simulink library "WaterRunner_lib"  (Simulink 7.9)
settings: Solver=ode45  StartTime=0.0  StopTime=10.0  RelTol=1e-3
values from neighbouring files (symbols this model uses):
  water_level = u(6)    [water_model.m]
undefined symbols (not defined in the file or in its folder): frame_inertia, frame_mass, initRobHeight, L2_inertia, L2_mass, L3_inertia, L3_mass, L4_inertia, L4_mass, median_speed, motor_inertia, motor_mass, mu_slide, mu_stick, phase_delay, pulse_amplitude, pulse_df, pulse_period, speed, switch_angle, Tail_inertia, Tail_mass, tau, V_H
libraries: mblibv1 x42, simulink x2
settings Model: Creator=Metti  LastModifiedBy=nitisht

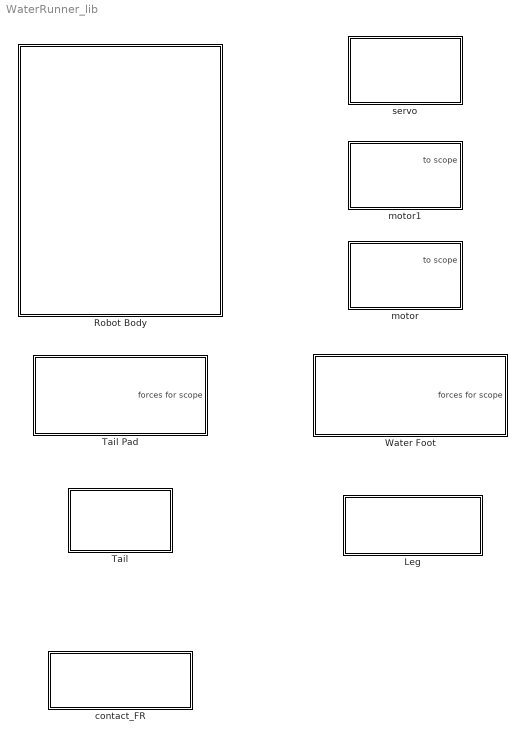
== system WaterRunner_lib ==
  Leg : Subsystem
      mask Description: mask for leg
  Robot Body : Subsystem  mask{initRobHeight=initRobHeight}
      mask prompts: initRobHeight "height"
  Tail : Subsystem
  Tail Pad : Subsystem
  Water Foot : Subsystem
  contact_FR : Subsystem
  motor : Subsystem  mask{variableName=work, ic_angle=0}
      mask prompts: variableName "Variable Name for Work"; ic_angle "initial angle"
      mask init:
      | set_param([gcb '/To Workspace'],'VariableName',variableName)
  motor1 : Subsystem  mask{speed=speed, X0=0, VariableName=work}
      mask prompts: speed "Rotation Speed:"; X0 "Initial output:"; VariableName "Variable name for Work:"
  servo : Subsystem  mask{tail_angle=speed, VariableName=work}
      mask prompts: tail_angle "Tail angle"; VariableName "Variable name for Work:"

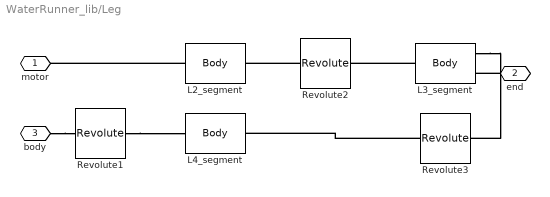
== system WaterRunner_lib/Leg ==
  L2_segment : mblibv1/Bodies/Body  LConnTagsString=CS1  RConnTagsString=CS2  UpdateFromCAD=off  DialogClass=MechanicalBodyBlock  Mass=L2_mass  MassUnits=kg  InertiaUnits=kg*m^2  Inertia=L2_inertia  Shape=Cylinder  ShapeDims=[1 1]  ShapeUnits=m  ShapeUse=false  Density=1  DensityUnits=kg/m^3  DensityUse=false  GraphicsMode=CONVHULL  BodyColorSelMode=COLORPALETTE  BodyColor=[0 0 0]  AttachedToCS=CG  CG=Left$CG$L2_CG$CS1$CS1$m$[0 0 0]$Euler X-Y-Z$deg$WORLD$false$none  WorkingFrames=Left$CS1$L2_CS1$Adjoining$Adjoining$m$[0 0 0]$Euler X-Y-Z$deg$WORLD$true$none#Right$CS2$L2_CS2$CS1$CS1$m$[0 0 0]$Euler X-Y-Z$deg$WORLD$true$none  CGPos=L2_CG  CGRot=[0 0 0]  CS0Pos=[]  CS0Rot=[]  CS1Pos=L2_CS1  CS1Rot=[0 0 0]  CS2Pos=L2_CS2  CS2Rot=[0 0 0]  CS3Pos=[]  CS3Rot=[]  CS4Pos=[]  CS4Rot=[]  CS5Pos=[]  CS5Rot=[]  CS6Pos=[]  CS6Rot=[]  CS7Pos=[]  CS7Rot=[]  CS8Pos=[]  CS8Rot=[]  CS9Pos=[]  CS9Rot=[]  CS10Pos=[]  CS10Rot=[]  CS11Pos=[]  CS11Rot=[]  CS12Pos=[]  CS12Rot=[]  CS13Pos=[]  CS13Rot=[]  CS14Pos=[]  CS14Rot=[]  CS15Pos=[]  CS15Rot=[]  CS16Pos=[]  CS16Rot=[]  CS17Pos=[]  CS17Rot=[]  CS18Pos=[]  CS18Rot=[]  CS19Pos=[]  CS19Rot=[]  CS20Pos=[]  CS20Rot=[]
  L3_segment : mblibv1/Bodies/Body  LConnTagsString=CS1  RConnTagsString=CS2|CS3  UpdateFromCAD=off  DialogClass=MechanicalBodyBlock  Mass=L3_mass  MassUnits=kg  InertiaUnits=kg*m^2  Inertia=L3_inertia  Shape=Cylinder  ShapeDims=[1 1]  ShapeUnits=m  ShapeUse=false  Density=1  DensityUnits=kg/m^3  DensityUse=false  GraphicsMode=CONVHULL  BodyColorSelMode=COLORPALETTE  BodyColor=[0 0 0]  AttachedToCS=CG  CG=Left$CG$L3_CG$CS1$CS1$m$[0 0 0]$Euler X-Y-Z$rad$CS1$false$none  WorkingFrames=Left$CS1$L3_CS1$Adjoining$Adjoining$m$L3_ori$Euler X-Y-Z$rad$Adjoining$true$none#Right$CS2$L3_CS2$CS1$CS1$m$[0 0 0]$Euler X-Y-Z$rad$CS1$true$none#Right$CS3$L3_CS3$CS1$CS1$m$[0 0 0]$Euler X-Y-Z$rad$CS1$true$none  CGPos=L3_CG  CGRot=[0 0 0]  CS0Pos=[]  CS0Rot=[]  CS1Pos=L3_CS1  CS1Rot=L3_ori  CS2Pos=L3_CS2  CS2Rot=[0 0 0]  CS3Pos=L3_CS3  CS3Rot=[0 0 0]  CS4Pos=[]  CS4Rot=[]  CS5Pos=[]  CS5Rot=[]  CS6Pos=[]  CS6Rot=[]  CS7Pos=[]  CS7Rot=[]  CS8Pos=[]  CS8Rot=[]  CS9Pos=[]  CS9Rot=[]  CS10Pos=[]  CS10Rot=[]  CS11Pos=[]  CS11Rot=[]  CS12Pos=[]  CS12Rot=[]  CS13Pos=[]  CS13Rot=[]  CS14Pos=[]  CS14Rot=[]  CS15Pos=[]  CS15Rot=[]  CS16Pos=[]  CS16Rot=[]  CS17Pos=[]  CS17Rot=[]  CS18Pos=[]  CS18Rot=[]  CS19Pos=[]  CS19Rot=[]  CS20Pos=[]  CS20Rot=[]
  L4_segment : mblibv1/Bodies/Body  LConnTagsString=CS1  RConnTagsString=CS2  UpdateFromCAD=off  DialogClass=MechanicalBodyBlock  Mass=L4_mass  MassUnits=kg  InertiaUnits=kg*m^2  Inertia=L4_inertia  Shape=Cylinder  ShapeDims=[1 1]  ShapeUnits=m  ShapeUse=false  Density=1  DensityUnits=kg/m^3  DensityUse=false  GraphicsMode=CONVHULL  BodyColorSelMode=COLORPALETTE  BodyColor=[0 0 0]  AttachedToCS=CG  CG=Left$CG$L4_CG$CS1$CS1$m$[0 0 0]$Euler X-Y-Z$rad$CS1$false$none  WorkingFrames=Left$CS1$L4_CS1$Adjoining$Adjoining$m$L4_ori$Euler X-Y-Z$rad$Adjoining$true$none#Right$CS2$L4_CS2$CS1$CS1$m$[0 0 0]$Euler X-Y-Z$rad$CS1$true$none  CGPos=L4_CG  CGRot=[0 0 0]  CS0Pos=[]  CS0Rot=[]  CS1Pos=L4_CS1  CS1Rot=L4_ori  CS2Pos=L4_CS2  CS2Rot=[0 0 0]  CS3Pos=[]  CS3Rot=[]  CS4Pos=[]  CS4Rot=[]  CS5Pos=[]  CS5Rot=[]  CS6Pos=[]  CS6Rot=[]  CS7Pos=[]  CS7Rot=[]  CS8Pos=[]  CS8Rot=[]  CS9Pos=[]  CS9Rot=[]  CS10Pos=[]  CS10Rot=[]  CS11Pos=[]  CS11Rot=[]  CS12Pos=[]  CS12Rot=[]  CS13Pos=[]  CS13Rot=[]  CS14Pos=[]  CS14Rot=[]  CS15Pos=[]  CS15Rot=[]  CS16Pos=[]  CS16Rot=[]  CS17Pos=[]  CS17Rot=[]  CS18Pos=[]  CS18Rot=[]  CS19Pos=[]  CS19Rot=[]  CS20Pos=[]  CS20Rot=[]
  Revolute1 : mblibv1/Joints/Revolute  LConnTagsString=__newl0  RConnTagsString=__newr0  UpdateFromCAD=off  NumSAPorts=0  CutJoint=off  MarkAsCut=off  Primitives=prismatic  PrimitiveProps=R1$WORLD$[0 0 1]$revolute  DialogClass=JointBlock  R1Axis=[0 0 1]
  Revolute2 : mblibv1/Joints/Revolute  LConnTagsString=__newl0  RConnTagsString=__newr0  UpdateFromCAD=off  NumSAPorts=0  CutJoint=off  MarkAsCut=off  Primitives=prismatic  PrimitiveProps=R1$WORLD$[0 0 1]$revolute  DialogClass=JointBlock  R1Axis=[0 0 1]
  Revolute3 : mblibv1/Joints/Revolute  LConnTagsString=__newl0  RConnTagsString=__newr0  UpdateFromCAD=off  NumSAPorts=0  CutJoint=on  MarkAsCut=off  Primitives=prismatic  PrimitiveProps=R1$World$[0 0 1]$revolute  DialogClass=JointBlock  R1Axis=[0 0 1]
  motor : PMIOPort  Port=1  Side=Left
  end : PMIOPort  Port=2  Side=Right
  body : PMIOPort  Port=3  Side=Left
  connections:
  body/RConn1 -- Revolute1/LConn1
  end/RConn1 -- L3_segment/RConn2
  Revolute3/LConn1 -- L4_segment/RConn1
  Revolute1/RConn1 -- L4_segment/LConn1
  L3_segment/RConn1 -- Revolute3/RConn1
  L3_segment/LConn1 -- Revolute2/RConn1
  Revolute2/LConn1 -- L2_segment/RConn1
  L2_segment/LConn1 -- motor/RConn1

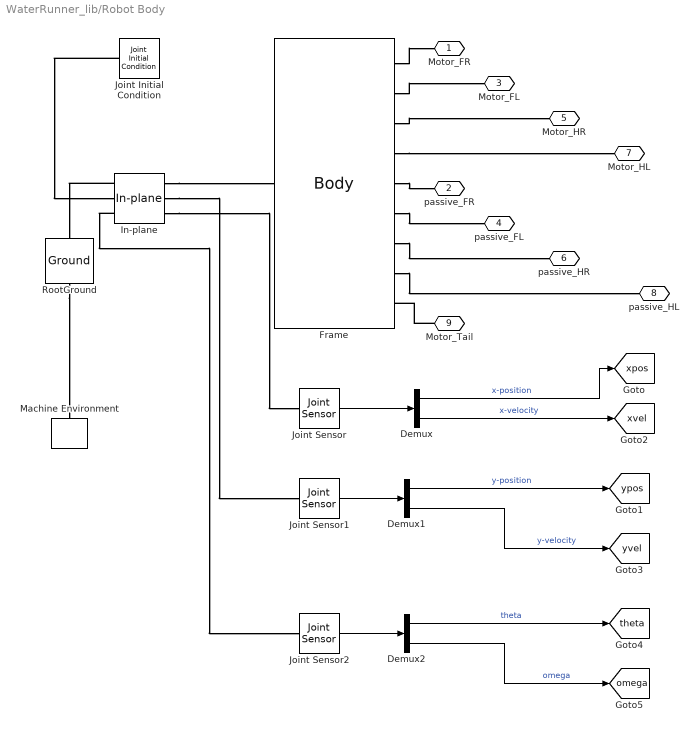
== system WaterRunner_lib/Robot Body ==
  Demux : Demux  Outputs=2
  Demux1 : Demux  Outputs=2
  Demux2 : Demux  Outputs=2
  Frame : mblibv1/Bodies/Body  LConnTagsString=CS1  RConnTagsString=CS6|CS7|CS8|CS9|CS10|CS11|CS12|CS13|CS14  UpdateFromCAD=off  DialogClass=MechanicalBodyBlock  Mass=frame_mass  MassUnits=kg  InertiaUnits=kg*m^2  Inertia=frame_inertia  Shape=Cylinder  ShapeDims=[1 1]  ShapeUnits=m  ShapeUse=false  Density=1  DensityUnits=kg/m^3  DensityUse=false  GraphicsMode=CONVHULL  BodyColorSelMode=COLORPALETTE  BodyColor=[0 0 1]  AttachedToCS=CG  CG=Left$CG$frame_CG$WORLD$WORLD$m$[0 0 0]$Euler X-Y-Z$deg$WORLD$false$none  WorkingFrames=Left$CS1$frame_CA$World$World$m$[0 0 0]$Euler X-Y-Z$deg$WORLD$true$none#Right$CS2$frame_FR$World$World$m$[0 0 0]$Euler X-Y-Z$deg$WORLD$false$none#Right$CS4$frame_FL$World$World$m$[0 0 0]$Euler X-Y-Z$deg$WORLD$false$none#Right$CS3$frame_HR$World$World$m$[0 0 0]$Euler X-Y-Z$deg$WORLD$false$none#Right$CS5$frame_HL$WORLD$WORLD$m$[0 0 0]$Euler X-Y-Z$deg$WORLD$false$none#Right$CS6$frame_motor_FR$WORLD$WORLD$m$[0 0 0]$Euler X-Y-Z$deg$WORLD$true$none#Right$CS7$frame_motor_FL$WORLD$WORLD$m$[0 0 0]$Euler X-Y-Z$deg$WORLD$true$none#Right$CS8$frame_motor_HR$WORLD$WORLD$m$[0 0 0]$Euler X-Y-Z$deg$WORLD$true$none#Right$CS9$frame_motor_HL$WORLD$WORLD$m$[0 0 0]$Euler X-Y-Z$deg$WORLD$true$none#Right$CS10$frame_passive_FR$WORLD$WORLD$m$[0 0 0]$Euler X-Y-Z$deg$WORLD$true$none#Right$CS11$frame_passive_FL$WORLD$WORLD$m$[0 0 0]$Euler X-Y-Z$deg$WORLD$true$none#Right$CS12$frame_passive_HR$WORLD$WORLD$m$[0 0 0]$Euler X-Y-Z$deg$WORLD$true$none#Right$CS13$frame_passive_HL$WORLD$WORLD$m$[0 0 0]$Euler X-Y-Z$deg$WORLD$true$none#Right$CS14$frame_motor_Tail$WORLD$WORLD$m$[0 0 0]$Euler X-Y-Z$deg$WORLD$true$none  CGPos=frame_CG  CGRot=[0 0 0]  CS0Pos=[]  CS0Rot=[]  CS1Pos=frame_CA  CS1Rot=[0 0 0]  CS2Pos=frame_FR  CS2Rot=[0 0 0]  CS3Pos=frame_HR  CS3Rot=[0 0 0]  CS4Pos=frame_FL  CS4Rot=[0 0 0]  CS5Pos=frame_HL  CS5Rot=[0 0 0]  CS6Pos=frame_motor_FR  CS6Rot=[0 0 0]  CS7Pos=frame_motor_FL  CS7Rot=[0 0 0]  CS8Pos=frame_motor_HR  CS8Rot=[0 0 0]  CS9Pos=frame_motor_HL  CS9Rot=[0 0 0]  CS10Pos=frame_passive_FR  CS10Rot=[0 0 0]  CS11Pos=frame_passive_FL  CS11Rot=[0 0 0]  CS12Pos=frame_passive_HR  CS12Rot=[0 0 0]  CS13Pos=frame_passive_HL  CS13Rot=[0 0 0]  CS14Pos=frame_motor_Tail  CS14Rot=[0 0 0]  CS15Pos=[]  CS15Rot=[]  CS16Pos=[]  CS16Rot=[]  CS17Pos=[]  CS17Rot=[]  CS18Pos=[]  CS18Rot=[]  CS19Pos=[]  CS19Rot=[]  CS20Pos=[]  CS20Rot=[]
  In-plane : mblibv1/Joints/In-plane  LConnTagsString=__newl0|SA1|SA2  RConnTagsString=__newr0|SA1|SA2  UpdateFromCAD=off  NumSAPorts=4  CutJoint=off  MarkAsCut=off  Primitives=prismatic  PrimitiveProps=P1$World$[1 0 0]$prismatic#P2$World$[0 1 0]$prismatic  DialogClass=JointBlock  P1Axis=[1 0 0]  P2Axis=[0 1 0]
  Joint Initial Condition : mblibv1/Sensors &  Actuators/Joint Initial Condition  UpdateFromCAD=off  LeftPortType=blob  RightPortType=blob  PhysicalDomain=mechanical  DialogClass=InitialConditionBlock  InitialConditions=P1$true$0$m$deg$0$m/s$deg/s#P2$true$initRobHeight$m$deg$0$m/s$deg/s#P3$false$0$m$deg$0$m/s$deg/s#R1$false$0$m$rad$0$m/s$rad/s#R2$false$0$m$deg$0$m/s$deg/s#R3$false$0$m$deg$0$m/s$deg/s#S$false$0$m$deg$0$m/s$deg/s  P1PIC=0  P1VIC=0  P2PIC=initRobHeight  P2VIC=0  P3PIC=0  P3VIC=0  R1PIC=0  R1VIC=0  R2PIC=0  R2VIC=0  R3PIC=0  R3VIC=0  SPIC=0  SVIC=0
  Joint Sensor : mblibv1/Sensors &  Actuators/Joint Sensor  UpdateFromCAD=off  PhysicalDomain=Mechanical  PortType=blob  Muxed=on  Pose=off  Angle=on  AngleUnits=deg  ArcVelocity=off  ArcVelocityUnits=deg/s  ArcAcceleration=off  ArcAccelerationUnits=deg/s^2  CoordPosition=on  CoordPositionUnits=m  Velocity=on  VelocityUnits=m/s  Acceleration=off  AccelerationUnits=m/s^2  Quaternion=on  QuaternionDT=off  QuaternionDDT=off  QuaternionUnits=off  OutputVector=[1]  ActiveIO=off  Width=2  DialogClass=MechanicalSensorBlock  Primitive=P1  Force=off  ForceUnits=N  Torque=off  TorqueUnits=N*m  ReferenceFrame=Absolute (World)  ReactionSensedSide=Base  ReactionReferenceFrame=Absolute (World)  ReactionForce=off  ReactionForceUnits=N  ReactionMoment=off  ReactionMomentUnits=N*m
  Joint Sensor1 : mblibv1/Sensors &  Actuators/Joint Sensor  UpdateFromCAD=off  PhysicalDomain=Mechanical  PortType=blob  Muxed=on  Pose=off  Angle=on  AngleUnits=deg  ArcVelocity=off  ArcVelocityUnits=deg/s  ArcAcceleration=off  ArcAccelerationUnits=deg/s^2  CoordPosition=on  CoordPositionUnits=m  Velocity=on  VelocityUnits=m/s  Acceleration=off  AccelerationUnits=m/s^2  Quaternion=on  QuaternionDT=off  QuaternionDDT=off  QuaternionUnits=off  OutputVector=[1]  ActiveIO=off  Width=2  DialogClass=MechanicalSensorBlock  Primitive=P2  Force=off  ForceUnits=N  Torque=off  TorqueUnits=N*m  ReferenceFrame=Absolute (World)  ReactionSensedSide=Base  ReactionReferenceFrame=Absolute (World)  ReactionForce=off  ReactionForceUnits=N  ReactionMoment=off  ReactionMomentUnits=N*m
  Joint Sensor2 : mblibv1/Sensors &  Actuators/Joint Sensor  UpdateFromCAD=off  PhysicalDomain=Mechanical  PortType=blob  Muxed=on  Pose=off  Angle=on  AngleUnits=rad  ArcVelocity=on  ArcVelocityUnits=rad/s  ArcAcceleration=off  ArcAccelerationUnits=deg/s^2  CoordPosition=on  CoordPositionUnits=m  Velocity=on  VelocityUnits=m/s  Acceleration=off  AccelerationUnits=m/s^2  Quaternion=on  QuaternionDT=off  QuaternionDDT=off  QuaternionUnits=off  OutputVector=[1]  ActiveIO=off  Width=1  DialogClass=MechanicalSensorBlock  Primitive=P2  Force=off  ForceUnits=N  Torque=off  TorqueUnits=N*m  ReferenceFrame=Absolute (World)  ReactionSensedSide=Base  ReactionReferenceFrame=Absolute (World)  ReactionForce=off  ReactionForceUnits=N  ReactionMoment=off  ReactionMomentUnits=N*m
  Machine Environment : mblibv1/Bodies/Machine Environment  PortType=env  PhysicalDomain=Mechanical  DialogTemplateClass=MECH.MachineEnvironment  SyncWhenCopied=off  Gravity=[0 -9.81 0]  GravityUnits=m/s^2  GravityAsSignal=off  Dimensionality=Auto-detect  AnalysisType=Forward dynamics  LinearAssemblyTolerance=1e-3  LinearAssemblyToleranceUnits=m  AngularAssemblyTolerance=1e-3  AngularAssemblyToleranceUnits=rad  ConstraintSolverType=Stabilizing  ConstraintRelTolerance=1e-4  ConstraintAbsTolerance=1e-4  UseRobustSingularityHandling=off  RedundancyAnalysisToleranceType=Automatically select tolerance  RedundancyAnalysisTolerance=1e-14  StatePerturbationType=Fixed  PerturbationSize=1e-5  VisualizeMachine=on  BodyVisualizationType=Use model default body geometries  BodyColorSelMode=Use model default  DefaultBodyColor=[1 0 0]
  RootGround : mblibv1/Bodies/Ground  UpdateFromCAD=on  LeftPortType=env  RightPortType=workingframe  PhysicalDomain=Mechanical  DialogClass=GroundBlock  CoordPosition=[0 0 0]  CoordPositionUnits=m  StateVectorMgrId=-1  MachineId=[0 0]  ShowEnvPort=on
  Motor_FR : PMIOPort  Port=1  Side=Right
  passive_FR : PMIOPort  Port=2  Side=Right
  Motor_FL : PMIOPort  Port=3  Side=Left
  passive_FL : PMIOPort  Port=4  Side=Left
  Motor_HR : PMIOPort  Port=5  Side=Right
  passive_HR : PMIOPort  Port=6  Side=Right
  Motor_HL : PMIOPort  Port=7  Side=Left
  passive_HL : PMIOPort  Port=8  Side=Left
  Motor_Tail : PMIOPort  Port=9  Side=Left
  tag scope: omega=global, theta=global, xpos=global, xvel=global, ypos=global, yvel=global
  wires:
  Joint Sensor/1 -> Demux/1
  Joint Sensor1/1 -> Demux1/1
  Demux/1 -> [xpos]  "x-position"
  Demux/2 -> [xvel]  "x-velocity"
  Demux1/1 -> [ypos]  "y-position"
  Demux1/2 -> [yvel]  "y-velocity"
  Demux2/1 -> [theta]  "theta"
  Demux2/2 -> [omega]  "omega"
  Joint Sensor2/1 -> Demux2/1
  connections:
  In-plane/RConn1 -- Frame/LConn1
  RootGround/LConn1 -- Machine Environment/RConn1
  In-plane/LConn1 -- RootGround/RConn1
  Frame/RConn1 -- Motor_FR/RConn1
  Frame/RConn2 -- Motor_FL/RConn1
  Frame/RConn3 -- Motor_HR/RConn1
  Frame/RConn4 -- Motor_HL/RConn1
  Frame/RConn5 -- passive_FR/RConn1
  Frame/RConn6 -- passive_FL/RConn1
  Frame/RConn7 -- passive_HR/RConn1
  Frame/RConn8 -- passive_HL/RConn1
  Joint Initial Condition/RConn1 -- In-plane/LConn2
  In-plane/RConn2 -- Joint Sensor1/LConn1
  Motor_Tail/RConn1 -- Frame/RConn9
  In-plane/RConn3 -- Joint Sensor/LConn1
  In-plane/LConn3 -- Joint Sensor2/LConn1

== system WaterRunner_lib/Tail ==
  L2_segment : mblibv1/Bodies/Body  LConnTagsString=CS1  RConnTagsString=CS2  UpdateFromCAD=off  DialogClass=MechanicalBodyBlock  Mass=Tail_mass  MassUnits=kg  InertiaUnits=kg*m^2  Inertia=Tail_inertia  Shape=Cylinder  ShapeDims=[1 1]  ShapeUnits=m  ShapeUse=false  Density=1  DensityUnits=kg/m^3  DensityUse=false  GraphicsMode=CONVHULL  BodyColorSelMode=COLORPALETTE  BodyColor=[0 0 0]  AttachedToCS=CG  CG=Left$CG$Tail_CG$CS1$CS1$m$[0 0 0]$Euler X-Y-Z$deg$WORLD$false$none  WorkingFrames=Left$CS1$Tail_CS1$Adjoining$Adjoining$m$[0 0 0]$Euler X-Y-Z$deg$WORLD$true$none#Right$CS2$Tail_CS2$CS1$CS1$m$[0 0 0]$Euler X-Y-Z$deg$WORLD$true$none  CGPos=Tail_CG  CGRot=[0 0 0]  CS0Pos=[]  CS0Rot=[]  CS1Pos=Tail_CS1  CS1Rot=[0 0 0]  CS2Pos=Tail_CS2  CS2Rot=[0 0 0]  CS3Pos=[]  CS3Rot=[]  CS4Pos=[]  CS4Rot=[]  CS5Pos=[]  CS5Rot=[]  CS6Pos=[]  CS6Rot=[]  CS7Pos=[]  CS7Rot=[]  CS8Pos=[]  CS8Rot=[]  CS9Pos=[]  CS9Rot=[]  CS10Pos=[]  CS10Rot=[]  CS11Pos=[]  CS11Rot=[]  CS12Pos=[]  CS12Rot=[]  CS13Pos=[]  CS13Rot=[]  CS14Pos=[]  CS14Rot=[]  CS15Pos=[]  CS15Rot=[]  CS16Pos=[]  CS16Rot=[]  CS17Pos=[]  CS17Rot=[]  CS18Pos=[]  CS18Rot=[]  CS19Pos=[]  CS19Rot=[]  CS20Pos=[]  CS20Rot=[]
  motor : PMIOPort  Port=1  Side=Left
  end : PMIOPort  Port=2  Side=Right
  connections:
  motor/RConn1 -- L2_segment/LConn1
  L2_segment/RConn1 -- end/RConn1

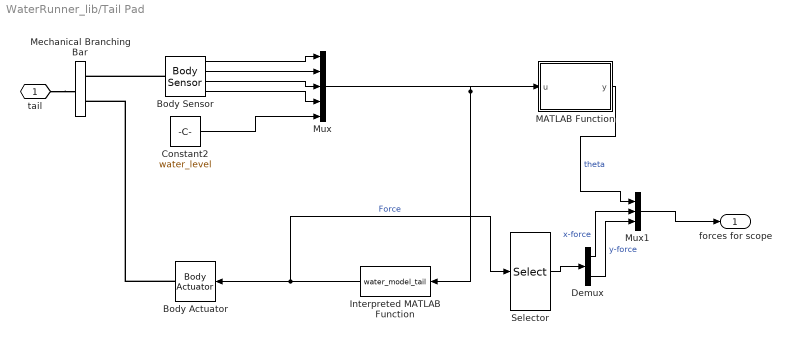
== system WaterRunner_lib/Tail Pad ==
  Body Actuator : mblibv1/Sensors &  Actuators/Body Actuator  UpdateFromCAD=off  PhysicalDomain=Mechanical  PortType=blob  ActuationStyle=Force  AngleUnits=deg  ArcVelocityUnits=deg/s  ArcAccelerationUnits=deg/s^2  CoordPositionUnits=m  VelocityUnits=m/s  AccelerationUnits=m/s^2  ForceUnits=N  TorqueUnits=N*m  ActiveIO=off  Width=6  DialogClass=MechanicalActuatorBlock  ReferenceFrame=Absolute (World)  Angle=off  CoordPosition=on  Force=on  Torque=on
  Body Sensor : mblibv1/Sensors &  Actuators/Body Sensor  UpdateFromCAD=off  PhysicalDomain=Mechanical  PortType=blob  Muxed=off  Pose=on  Angle=on  AngleUnits=deg  ArcVelocity=on  ArcVelocityUnits=rad/s  ArcAcceleration=off  ArcAccelerationUnits=deg/s^2  CoordPosition=on  CoordPositionUnits=m  Velocity=on  VelocityUnits=m/s  Acceleration=off  AccelerationUnits=m/s^2  Quaternion=on  QuaternionDT=off  QuaternionDDT=off  QuaternionUnits=off  OutputVector=[1]  ActiveIO=off  Width=18  DialogClass=MechanicalSensorBlock  ReferenceFrame=Absolute (World)
  Constant2 : Constant  Value=water_level
  Demux : Demux  Outputs=2
  Interpreted MATLAB Function : MATLABFcn  MATLABFcn=water_model_tail
  MATLAB Function : MATLAB Function  TreatAsAtomicUnit=on
  Mechanical Branching Bar : mblibv1/Utilities/Mechanical Branching Bar  LConnTagsString=_newl0  RConnTagsString=__newr0|SA2  UpdateFromCAD=off  DialogClass=MechanicalBranchingBarBlock  NumSAPorts=2
  Mux : Mux  Inputs=5
  Mux1 : Mux  Inputs=3
  Selector : Selector  InputPortWidth=6  IndexOptions=Index vector (dialog)  Indices=[4 5]  OutputSizes=1
  tail : PMIOPort  Port=1  Side=Left
  forces for scope : Outport
  wires:
  Demux/2 -> Mux1/3  "y-force"
  Demux/1 -> Mux1/2  "x-force"
  Selector/1 -> Demux/1
  Mux1/1 -> forces for scope/1
  MATLAB Function/1(y) -> Mux1/1  "theta"
  Interpreted MATLAB Function/1 -> Selector/1, Body Actuator/1  "Force"
  Constant2/1 -> Mux/5
  Body Sensor/4 -> Mux/4
  Body Sensor/3 -> Mux/3
  Body Sensor/2 -> Mux/2
  Body Sensor/1 -> Mux/1
  Mux/1 -> MATLAB Function/1(u), Interpreted MATLAB Function/1
  connections:
  Body Actuator/RConn1 -- Mechanical Branching Bar/RConn2
  Body Sensor/LConn1 -- Mechanical Branching Bar/RConn1
  tail/RConn1 -- Mechanical Branching Bar/LConn1

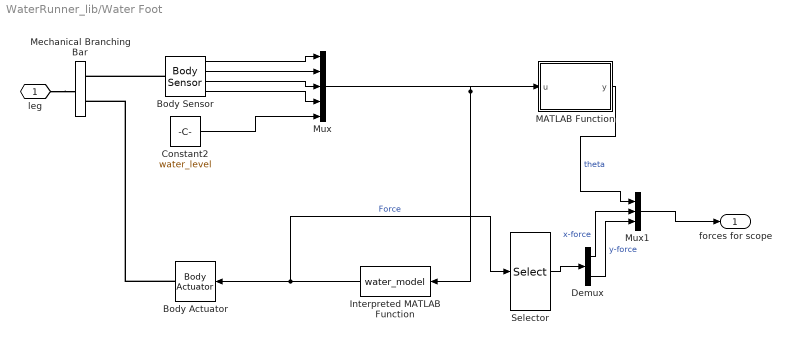
== system WaterRunner_lib/Water Foot ==
  Body Actuator : mblibv1/Sensors &  Actuators/Body Actuator  UpdateFromCAD=off  PhysicalDomain=Mechanical  PortType=blob  ActuationStyle=Force  AngleUnits=deg  ArcVelocityUnits=deg/s  ArcAccelerationUnits=deg/s^2  CoordPositionUnits=m  VelocityUnits=m/s  AccelerationUnits=m/s^2  ForceUnits=N  TorqueUnits=N*m  ActiveIO=off  Width=6  DialogClass=MechanicalActuatorBlock  ReferenceFrame=Absolute (World)  Angle=off  CoordPosition=on  Force=on  Torque=on
  Body Sensor : mblibv1/Sensors &  Actuators/Body Sensor  UpdateFromCAD=off  PhysicalDomain=Mechanical  PortType=blob  Muxed=off  Pose=on  Angle=on  AngleUnits=deg  ArcVelocity=on  ArcVelocityUnits=rad/s  ArcAcceleration=off  ArcAccelerationUnits=deg/s^2  CoordPosition=on  CoordPositionUnits=m  Velocity=on  VelocityUnits=m/s  Acceleration=off  AccelerationUnits=m/s^2  Quaternion=on  QuaternionDT=off  QuaternionDDT=off  QuaternionUnits=off  OutputVector=[1]  ActiveIO=off  Width=18  DialogClass=MechanicalSensorBlock  ReferenceFrame=Absolute (World)
  Constant2 : Constant  Value=water_level
  Demux : Demux  Outputs=2
  Interpreted MATLAB Function : MATLABFcn  MATLABFcn=water_model
  MATLAB Function : MATLAB Function  TreatAsAtomicUnit=on
  Mechanical Branching Bar : mblibv1/Utilities/Mechanical Branching Bar  LConnTagsString=_newl0  RConnTagsString=__newr0|SA2  UpdateFromCAD=off  DialogClass=MechanicalBranchingBarBlock  NumSAPorts=2
  Mux : Mux  Inputs=5
  Mux1 : Mux  Inputs=3
  Selector : Selector  InputPortWidth=6  IndexOptions=Index vector (dialog)  Indices=[4 5]  OutputSizes=1
  leg : PMIOPort  Port=1  Side=Left
  forces for scope : Outport
  wires:
  Demux/2 -> Mux1/3  "y-force"
  Demux/1 -> Mux1/2  "x-force"
  Selector/1 -> Demux/1
  Mux1/1 -> forces for scope/1
  MATLAB Function/1(y) -> Mux1/1  "theta"
  Interpreted MATLAB Function/1 -> Selector/1, Body Actuator/1  "Force"
  Constant2/1 -> Mux/5
  Body Sensor/4 -> Mux/4
  Body Sensor/3 -> Mux/3
  Body Sensor/2 -> Mux/2
  Body Sensor/1 -> Mux/1
  Mux/1 -> MATLAB Function/1(u), Interpreted MATLAB Function/1
  connections:
  Body Actuator/RConn1 -- Mechanical Branching Bar/RConn2
  Body Sensor/LConn1 -- Mechanical Branching Bar/RConn1
  leg/RConn1 -- Mechanical Branching Bar/LConn1

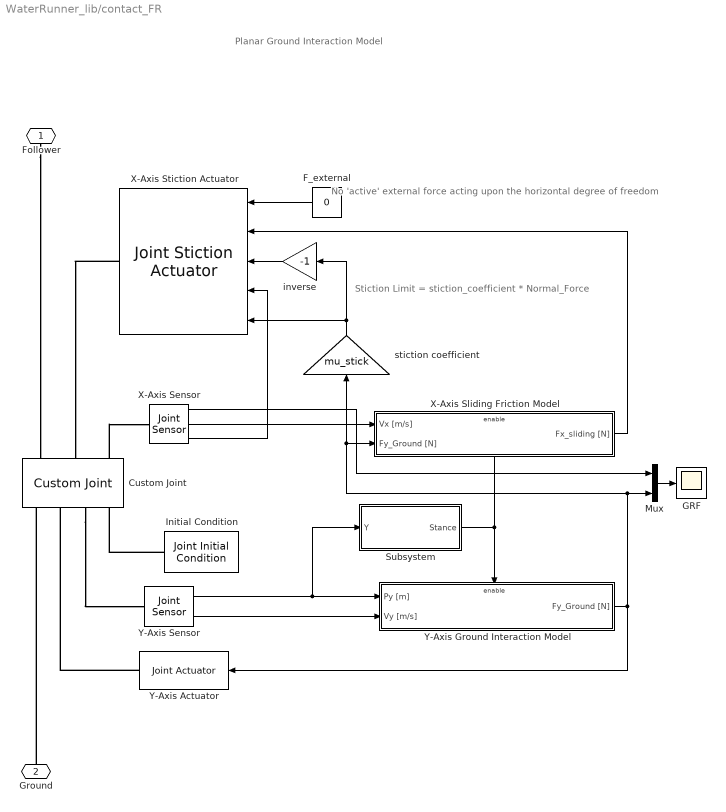
== system WaterRunner_lib/contact_FR ==
  note: Planar Ground Interaction Model
  note: No 'active' external force acting
      | upon the horizontal degree of freedom
  note: Stiction Limit
      | =
      | stiction_coefficient
      | *
      | Normal_Force
  Custom Joint : mblibv1/Joints/Custom Joint  LConnTagsString=__newl0|SA1|SA2|SA3  RConnTagsString=__newr0|SA1|SA2  UpdateFromCAD=off  NumSAPorts=5  CutJoint=off  MarkAsCut=off  Primitives=prismatic_prismatic_prismatic_revolute  PrimitiveProps=P1$WORLD$[1 0 0]$prismatic#P2$WORLD$[0 1 0]$prismatic#P3$WORLD$[0 0 1]$prismatic#R1$WORLD$[0 0 1]$revolute  DialogClass=JointBlock  R1Axis=[0 0 1]  R2Axis=[]  R3Axis=[]  P1Axis=[1 0 0]  P2Axis=[0 1 0]  P3Axis=[0 0 1]  SAxis=[]
  F_external : Constant  Value=0
  GRF : Scope
      settings: TimeRange=10  YMin=-1  YMax=19
  Initial Condition : mblibv1/Sensors &  Actuators/Joint Initial Condition  UpdateFromCAD=off  LeftPortType=blob  RightPortType=blob  PhysicalDomain=Mechanical  DialogClass=InitialConditionBlock  InitialConditions=P1$false$0$m$rad$0$m/s$rad/s#P2$false$0$m$rad$0$m/s$rad/s#P3$false$0$m$rad$0$m/s$rad/s#R1$false$0$m$rad$0$m/s$rad/s#R2$false$0$m$rad$0$m/s$rad/s#R3$false$0$m$rad$0$m/s$rad/s#S$false$0$m$rad$0$m/s$rad/s  P1PIC=0  P1VIC=0  P2PIC=0  P2VIC=0  P3PIC=0  P3VIC=0  R1PIC=0  R1VIC=0  R2PIC=0  R2VIC=0  R3PIC=0  R3VIC=0  SPIC=0  SVIC=0
  Mux : Mux  Inputs=2
  Subsystem : Subsystem
  X-Axis Sensor : mblibv1/Sensors &  Actuators/Joint Sensor  UpdateFromCAD=off  PhysicalDomain=Mechanical  PortType=blob  Muxed=off  Pose=off  Angle=on  AngleUnits=deg  ArcVelocity=off  ArcVelocityUnits=deg/s  ArcAcceleration=off  ArcAccelerationUnits=deg/s^2  CoordPosition=on  CoordPositionUnits=m  Velocity=on  VelocityUnits=m/s  Acceleration=off  AccelerationUnits=m/s^2  Quaternion=on  QuaternionDT=off  QuaternionDDT=off  QuaternionUnits=off  OutputVector=[ 1 1 1 ]  ActiveIO=off  Width=3  DialogClass=MechanicalSensorBlock  Primitive=P1  Force=on  ForceUnits=N  Torque=off  TorqueUnits=N-m  ReferenceFrame=Absolute (INERTIAL)  ReactionSensedSide=Base  ReactionReferenceFrame=Absolute (World)  ReactionForce=off  ReactionForceUnits=N  ReactionMoment=off  ReactionMomentUnits=N-m
  X-Axis Sliding Friction Model : Subsystem
  X-Axis Stiction Actuator : mblibv1/Sensors &  Actuators/Joint Stiction Actuator  UpdateFromCAD=off  PhysicalDomain=Mechanical  PortType=blob  ActuationStyle=Force  AngleUnits=deg  ArcVelocityUnits=deg/s  ArcAccelerationUnits=deg/s^2  CoordPositionUnits=m  VelocityUnits=m/s  AccelerationUnits=m/s^2  ForceUnits=N  TorqueUnits=N-m  ActiveIO=off  Width=5  DialogClass=EventActuatorBlock  Primitive=P1  FrictionalForceUnits=N  ExternalForceUnits=N  FrictionalTorqueUnits=N*m  ExternalTorqueUnits=N*m  LockingTolerance=1e-3
  Y-Axis Actuator : mblibv1/Sensors &  Actuators/Joint Actuator  UpdateFromCAD=off  PhysicalDomain=Mechanical  PortType=blob  ActuationStyle=Force  AngleUnits=deg  ArcVelocityUnits=deg/s  ArcAccelerationUnits=deg/s^2  CoordPositionUnits=m  VelocityUnits=m/s  AccelerationUnits=m/s^2  ForceUnits=N  TorqueUnits=N*m  ActiveIO=off  Width=1  DialogClass=MechanicalActuatorBlock  Primitive=P2  ReferenceFrame=Absolute (INERTIAL)
  Y-Axis Ground Interaction Model : Subsystem
  Y-Axis Sensor : mblibv1/Sensors &  Actuators/Joint Sensor  UpdateFromCAD=off  PhysicalDomain=Mechanical  PortType=blob  Muxed=off  Pose=off  Angle=on  AngleUnits=deg  ArcVelocity=off  ArcVelocityUnits=deg/s  ArcAcceleration=off  ArcAccelerationUnits=deg/s^2  CoordPosition=on  CoordPositionUnits=m  Velocity=on  VelocityUnits=m/s  Acceleration=off  AccelerationUnits=m/s^2  Quaternion=on  QuaternionDT=off  QuaternionDDT=off  QuaternionUnits=off  OutputVector=[ 1 1 ]  ActiveIO=off  Width=2  DialogClass=MechanicalSensorBlock  Primitive=P2  Force=off  ForceUnits=N  Torque=off  TorqueUnits=N*m  ReferenceFrame=Absolute (INERTIAL)  ReactionSensedSide=Base  ReactionReferenceFrame=Absolute (World)  ReactionForce=off  ReactionForceUnits=N  ReactionMoment=off  ReactionMomentUnits=N*m
  inverse : Gain  Gain=-1
  stiction coefficient : Gain  Gain=mu_stick
  Follower : PMIOPort  Port=1  Side=Right
  Ground : PMIOPort  Port=2  Side=Left
  wires:
  Y-Axis Sensor/2 -> Y-Axis Ground Interaction Model/2(Vy [m/s])
  Y-Axis Sensor/1 -> Y-Axis Ground Interaction Model/1(Py [m]), Subsystem/1(Y)
  Y-Axis Ground Interaction Model/1(Fy_Ground [N]) -> Y-Axis Actuator/1, X-Axis Sliding Friction Model/2(Fy_Ground [N]), stiction coefficient/1, Mux/2
  Subsystem/1(Stance) -> Y-Axis Ground Interaction Model/Enable, X-Axis Sliding Friction Model/Enable
  F_external/1 -> X-Axis Stiction Actuator/1
  X-Axis Sliding Friction Model/1(Fx_sliding [N]) -> X-Axis Stiction Actuator/2
  inverse/1 -> X-Axis Stiction Actuator/3
  stiction coefficient/1 -> inverse/1, X-Axis Stiction Actuator/5
  Mux/1 -> GRF/1
  X-Axis Sensor/3 -> X-Axis Stiction Actuator/4
  X-Axis Sensor/2 -> X-Axis Sliding Friction Model/1(Vx [m/s])
  X-Axis Sensor/1 -> Mux/1
  connections:
  Y-Axis Actuator/RConn1 -- Custom Joint/LConn2
  Custom Joint/LConn3 -- Y-Axis Sensor/LConn1
  X-Axis Stiction Actuator/RConn1 -- Custom Joint/RConn2
  Custom Joint/RConn3 -- X-Axis Sensor/LConn1
  Follower/RConn1 -- Custom Joint/RConn1
  Ground/RConn1 -- Custom Joint/LConn1
  Initial Condition/RConn1 -- Custom Joint/LConn4

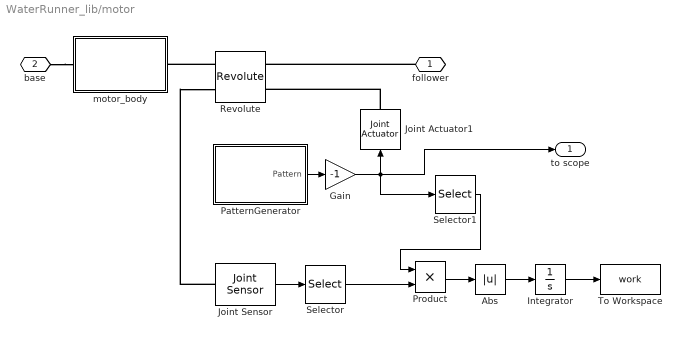
== system WaterRunner_lib/motor ==
  Abs : Abs
  Gain : Gain  Gain=-1
  Integrator : Integrator
  Joint Actuator1 : mblibv1/Sensors &  Actuators/Joint Actuator  UpdateFromCAD=off  PhysicalDomain=Mechanical  PortType=blob  ActuationStyle=Motion  AngleUnits=rad  ArcVelocityUnits=rad/s  ArcAccelerationUnits=rad/s^2  CoordPositionUnits=m  VelocityUnits=m/s  AccelerationUnits=m/s^2  ForceUnits=N  TorqueUnits=N*m  ActiveIO=off  Width=3  DialogClass=MechanicalActuatorBlock  Primitive=R1  ReferenceFrame=Absolute (World)
  Joint Sensor : mblibv1/Sensors &  Actuators/Joint Sensor  UpdateFromCAD=off  PhysicalDomain=Mechanical  PortType=blob  Muxed=off  Pose=off  Angle=off  AngleUnits=rad  ArcVelocity=off  ArcVelocityUnits=rad/s  ArcAcceleration=off  ArcAccelerationUnits=deg/s^2  CoordPosition=on  CoordPositionUnits=m  Velocity=off  VelocityUnits=m/s  Acceleration=off  AccelerationUnits=m/s^2  Quaternion=on  QuaternionDT=off  QuaternionDDT=off  QuaternionUnits=off  OutputVector=[1]  ActiveIO=off  Width=3  DialogClass=MechanicalSensorBlock  Primitive=R1  Force=off  ForceUnits=N  Torque=off  TorqueUnits=N*m  ReferenceFrame=Absolute (World)  ReactionSensedSide=Base  ReactionReferenceFrame=Absolute (World)  ReactionForce=off  ReactionForceUnits=N  ReactionMoment=on  ReactionMomentUnits=N*m
  PatternGenerator : Subsystem
  Product : Product  RndMeth=Zero
  Revolute : mblibv1/Joints/Revolute  LConnTagsString=__newl0|SA1  RConnTagsString=__newr0|SA1  UpdateFromCAD=off  NumSAPorts=2  CutJoint=off  MarkAsCut=off  Primitives=prismatic  PrimitiveProps=R1$World$[0 0 1]$revolute  DialogClass=JointBlock  R1Axis=[0 0 1]
  Selector : Selector  InputPortWidth=3  IndexOptions=Index vector (dialog)  Indices=[ 3]  OutputSizes=1
  Selector1 : Selector  InputPortWidth=3  IndexOptions=Index vector (dialog)  Indices=2  OutputSizes=1
  To Workspace : ToWorkspace  VariableName=work  SampleTime=-1  SaveFormat=Structure With Time
  motor_body : Subsystem
  follower : PMIOPort  Port=1  Side=Right
  base : PMIOPort  Port=2  Side=Left
  to scope : Outport
  wires:
  Product/1 -> Abs/1
  Abs/1 -> Integrator/1
  Integrator/1 -> To Workspace/1
  Joint Sensor/1 -> Selector/1
  Selector/1 -> Product/2
  Selector1/1 -> Product/1
  PatternGenerator/1(Pattern) -> Gain/1
  Gain/1 -> Joint Actuator1/1, Selector1/1, to scope/1
  connections:
  Revolute/LConn1 -- motor_body/RConn1
  follower/RConn1 -- Revolute/RConn1
  base/RConn1 -- motor_body/LConn1
  Joint Sensor/LConn1 -- Revolute/LConn2
  Joint Actuator1/RConn1 -- Revolute/RConn2

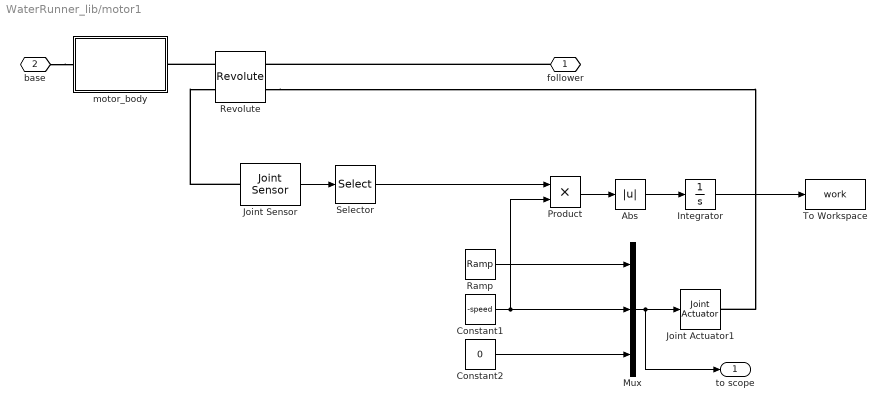
== system WaterRunner_lib/motor1 ==
  Abs : Abs
  Constant1 : Constant  Value=-speed
  Constant2 : Constant  Value=0
  Integrator : Integrator
  Joint Actuator1 : mblibv1/Sensors &  Actuators/Joint Actuator  UpdateFromCAD=off  PhysicalDomain=Mechanical  PortType=blob  ActuationStyle=Motion  AngleUnits=rad  ArcVelocityUnits=rad/s  ArcAccelerationUnits=rad/s^2  CoordPositionUnits=m  VelocityUnits=m/s  AccelerationUnits=m/s^2  ForceUnits=N  TorqueUnits=N*m  ActiveIO=off  Width=3  DialogClass=MechanicalActuatorBlock  Primitive=R1  ReferenceFrame=Absolute (World)
  Joint Sensor : mblibv1/Sensors &  Actuators/Joint Sensor  UpdateFromCAD=off  PhysicalDomain=Mechanical  PortType=blob  Muxed=off  Pose=off  Angle=off  AngleUnits=deg  ArcVelocity=off  ArcVelocityUnits=deg/s  ArcAcceleration=off  ArcAccelerationUnits=deg/s^2  CoordPosition=on  CoordPositionUnits=m  Velocity=off  VelocityUnits=m/s  Acceleration=off  AccelerationUnits=m/s^2  Quaternion=on  QuaternionDT=off  QuaternionDDT=off  QuaternionUnits=off  OutputVector=[1]  ActiveIO=off  Width=3  DialogClass=MechanicalSensorBlock  Primitive=R1  Force=off  ForceUnits=N  Torque=off  TorqueUnits=N*m  ReferenceFrame=Absolute (World)  ReactionSensedSide=Base  ReactionReferenceFrame=Absolute (World)  ReactionForce=off  ReactionForceUnits=N  ReactionMoment=on  ReactionMomentUnits=N*m
  Mux : Mux  Inputs=3
  Product : Product  RndMeth=Zero
  Ramp : simulink/Sources/Ramp  slope=-speed  start=0  X0=X0
  Revolute : mblibv1/Joints/Revolute  LConnTagsString=__newl0|SA1  RConnTagsString=__newr0|SA1  UpdateFromCAD=off  NumSAPorts=2  CutJoint=off  MarkAsCut=off  Primitives=prismatic  PrimitiveProps=R1$World$[0 0 1]$revolute  DialogClass=JointBlock  R1Axis=[0 0 1]
  Selector : Selector  InputPortWidth=3  IndexOptions=Index vector (dialog)  Indices=[ 3]  OutputSizes=1
  To Workspace : ToWorkspace  VariableName=work  SampleTime=-1  SaveFormat=Structure With Time
  motor_body : Subsystem
  follower : PMIOPort  Port=1  Side=Right
  base : PMIOPort  Port=2  Side=Left
  to scope : Outport
  wires:
  Mux/1 -> Joint Actuator1/1, to scope/1
  Constant2/1 -> Mux/3
  Constant1/1 -> Product/2, Mux/2
  Ramp/1 -> Mux/1
  Joint Sensor/1 -> Selector/1
  Selector/1 -> Product/1
  Abs/1 -> Integrator/1
  Product/1 -> Abs/1
  Integrator/1 -> To Workspace/1
  connections:
  Revolute/RConn2 -- Joint Actuator1/RConn1
  base/RConn1 -- motor_body/LConn1
  follower/RConn1 -- Revolute/RConn1
  Revolute/LConn1 -- motor_body/RConn1
  Joint Sensor/LConn1 -- Revolute/LConn2

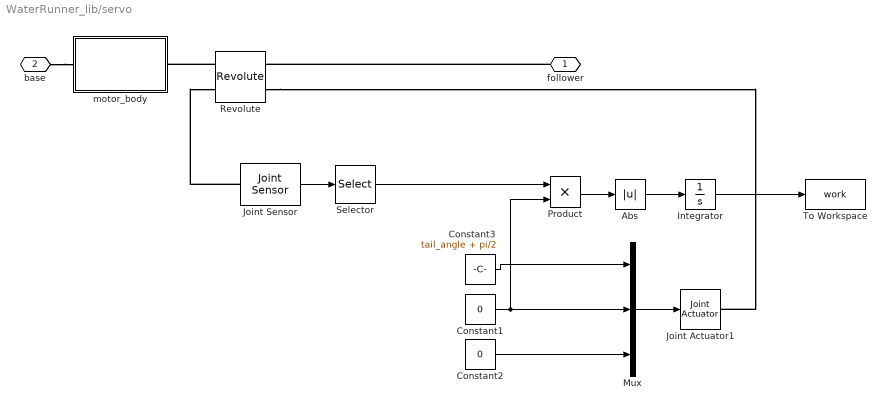
== system WaterRunner_lib/servo ==
  Abs : Abs
  Constant1 : Constant  Value=0
  Constant2 : Constant  Value=0
  Constant3 : Constant  Value=tail_angle + pi/2
  Integrator : Integrator
  Joint Actuator1 : mblibv1/Sensors &  Actuators/Joint Actuator  UpdateFromCAD=off  PhysicalDomain=Mechanical  PortType=blob  ActuationStyle=Motion  AngleUnits=rad  ArcVelocityUnits=rad/s  ArcAccelerationUnits=rad/s^2  CoordPositionUnits=m  VelocityUnits=m/s  AccelerationUnits=m/s^2  ForceUnits=N  TorqueUnits=N*m  ActiveIO=off  Width=3  DialogClass=MechanicalActuatorBlock  Primitive=R1  ReferenceFrame=Absolute (World)
  Joint Sensor : mblibv1/Sensors &  Actuators/Joint Sensor  UpdateFromCAD=off  PhysicalDomain=Mechanical  PortType=blob  Muxed=off  Pose=off  Angle=off  AngleUnits=deg  ArcVelocity=off  ArcVelocityUnits=deg/s  ArcAcceleration=off  ArcAccelerationUnits=deg/s^2  CoordPosition=on  CoordPositionUnits=m  Velocity=off  VelocityUnits=m/s  Acceleration=off  AccelerationUnits=m/s^2  Quaternion=on  QuaternionDT=off  QuaternionDDT=off  QuaternionUnits=off  OutputVector=[1]  ActiveIO=off  Width=3  DialogClass=MechanicalSensorBlock  Primitive=R1  Force=off  ForceUnits=N  Torque=off  TorqueUnits=N*m  ReferenceFrame=Absolute (World)  ReactionSensedSide=Base  ReactionReferenceFrame=Absolute (World)  ReactionForce=off  ReactionForceUnits=N  ReactionMoment=on  ReactionMomentUnits=N*m
  Mux : Mux  Inputs=3
  Product : Product  RndMeth=Zero
  Revolute : mblibv1/Joints/Revolute  LConnTagsString=__newl0|SA1  RConnTagsString=__newr0|SA1  UpdateFromCAD=off  NumSAPorts=2  CutJoint=off  MarkAsCut=off  Primitives=prismatic  PrimitiveProps=R1$World$[0 0 1]$revolute  DialogClass=JointBlock  R1Axis=[0 0 1]
  Selector : Selector  InputPortWidth=3  IndexOptions=Index vector (dialog)  Indices=[ 3]  OutputSizes=1
  To Workspace : ToWorkspace  VariableName=work  SampleTime=-1  SaveFormat=Structure With Time
  motor_body : Subsystem
  follower : PMIOPort  Port=1  Side=Right
  base : PMIOPort  Port=2  Side=Left
  wires:
  Mux/1 -> Joint Actuator1/1
  Constant2/1 -> Mux/3
  Constant1/1 -> Product/2, Mux/2
  Constant3/1 -> Mux/1
  Joint Sensor/1 -> Selector/1
  Selector/1 -> Product/1
  Abs/1 -> Integrator/1
  Product/1 -> Abs/1
  Integrator/1 -> To Workspace/1
  connections:
  Revolute/RConn2 -- Joint Actuator1/RConn1
  base/RConn1 -- motor_body/LConn1
  follower/RConn1 -- Revolute/RConn1
  Revolute/LConn1 -- motor_body/RConn1
  Joint Sensor/LConn1 -- Revolute/LConn2

== system WaterRunner_lib/contact_FR/Subsystem ==
  Y : Inport
  Fcn2 : Fcn  Expr=u<0
  Stance : Outport
  wires:
  Y/1 -> Fcn2/1
  Fcn2/1 -> Stance/1

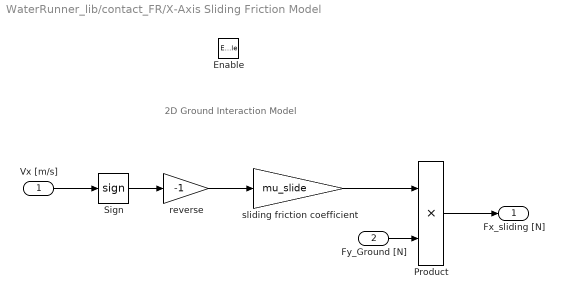
== system WaterRunner_lib/contact_FR/X-Axis Sliding Friction Model ==
  note: 2D Ground Interaction Model
  Vx [m/s] : Inport
  Fy_Ground [N] : Inport  Port=2
  Enable : EnablePort  StatesWhenEnabling=reset  PropagateVarSize=During execution  ZeroCross=off
  Product : Product  RndMeth=Zero
  Sign : Signum
  reverse : Gain  Gain=-1
  sliding friction coefficient : Gain  Gain=mu_slide
  Fx_sliding [N] : Outport  OutputWhenDisabled=reset  InitialOutput=0
      settings: AttributesFormatString=initial = '%<InitialOutput>'\nwhen disabled = '%<OutputWhenDisabled>'
  wires:
  Vx [m/s]/1 -> Sign/1
  Sign/1 -> reverse/1
  reverse/1 -> sliding friction coefficient/1
  Product/1 -> Fx_sliding [N]/1
  sliding friction coefficient/1 -> Product/1
  Fy_Ground [N]/1 -> Product/2

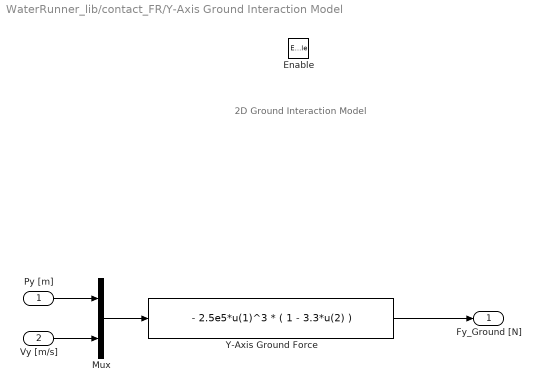
== system WaterRunner_lib/contact_FR/Y-Axis Ground Interaction Model ==
  note: 2D Ground Interaction Model
  Py [m] : Inport
  Vy [m/s] : Inport  Port=2
  Enable : EnablePort  StatesWhenEnabling=reset  PropagateVarSize=During execution  ZeroCross=off
  Mux : Mux  Inputs=2
  Y-Axis Ground Force : Fcn  Expr=- 2.5e5*u(1)^3 * ( 1 - 3.3*u(2) )
  Fy_Ground [N] : Outport  OutputWhenDisabled=reset  InitialOutput=0
      settings: AttributesFormatString=initial = '%<InitialOutput>'\nwhen disabled = '%<OutputWhenDisabled>'
  wires:
  Mux/1 -> Y-Axis Ground Force/1
  Py [m]/1 -> Mux/1
  Vy [m/s]/1 -> Mux/2
  Y-Axis Ground Force/1 -> Fy_Ground [N]/1

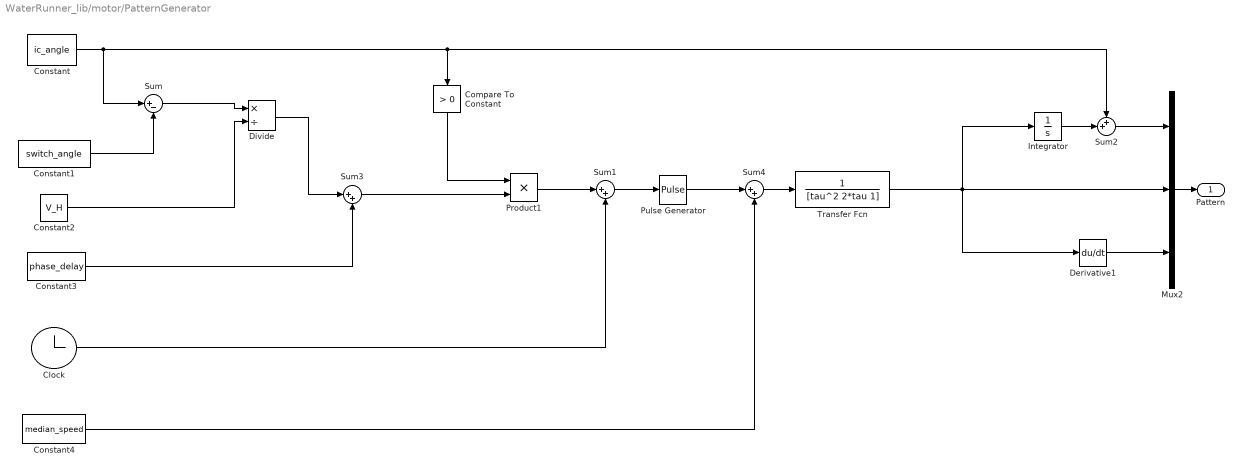
== system WaterRunner_lib/motor/PatternGenerator ==
  Clock : Clock
  Compare To Constant : simulink/Logic and Bit Operations/Compare To Constant  relop=>  const=0  OutDataTypeStr=uint8
  Constant : Constant  Value=ic_angle
  Constant1 : Constant  Value=switch_angle
  Constant2 : Constant  Value=V_H
  Constant3 : Constant  Value=phase_delay
  Constant4 : Constant  Value=median_speed
  Derivative1 : Derivative
  Divide : Product  Inputs=*/  RndMeth=Zero
  Integrator : Integrator
  Mux2 : Mux  Inputs=3
  Product1 : Product  RndMeth=Zero
  Pulse Generator : DiscretePulseGenerator  PulseType=Time based  TimeSource=Use external signal  Amplitude=pulse_amplitude  Period=pulse_period  PulseWidth=pulse_df  PhaseDelay=phase_delay
  Sum : Sum  Inputs=|+-
  Sum1 : Sum  Inputs=|++
  Sum2 : Sum  Inputs=++|
  Sum3 : Sum  Inputs=|++
  Sum4 : Sum  Inputs=|++
  Transfer Fcn : TransferFcn  Denominator=[tau^2 2*tau 1]
  Pattern : Outport
  wires:
  Clock/1 -> Sum1/2
  Sum1/1 -> Pulse Generator/1
  Mux2/1 -> Pattern/1
  Derivative1/1 -> Mux2/3
  Integrator/1 -> Sum2/2
  Sum2/1 -> Mux2/1
  Constant/1 -> Sum/1, Sum2/1, Compare To Constant/1
  Constant1/1 -> Sum/2
  Sum/1 -> Divide/1
  Constant3/1 -> Sum3/2
  Divide/1 -> Sum3/1
  Sum3/1 -> Product1/2
  Compare To Constant/1 -> Product1/1
  Product1/1 -> Sum1/1
  Constant2/1 -> Divide/2
  Pulse Generator/1 -> Sum4/1
  Constant4/1 -> Sum4/2
  Sum4/1 -> Transfer Fcn/1
  Transfer Fcn/1 -> Mux2/2, Integrator/1, Derivative1/1

== system WaterRunner_lib/motor/motor_body ==
  Body1 : mblibv1/Bodies/Body  LConnTagsString=CS1  RConnTagsString=CS2  UpdateFromCAD=off  DialogClass=MechanicalBodyBlock  Mass=motor_mass  MassUnits=kg  InertiaUnits=kg*m^2  Inertia=motor_inertia  Shape=Cylinder  ShapeDims=[1 1]  ShapeUnits=m  ShapeUse=false  Density=1  DensityUnits=kg/m^3  DensityUse=false  GraphicsMode=CONVHULL  BodyColorSelMode=COLORPALETTE  BodyColor=[0.87059 0.4902 0]  AttachedToCS=CG  CG=Left$CG$[0 0 0]$CS1$CS1$m$[0 0 0]$Euler X-Y-Z$deg$WORLD$false$none  WorkingFrames=Left$CS1$[0 0 0]$Adjoining$Adjoining$m$[0 0 0]$Euler X-Y-Z$deg$WORLD$true$none#Right$CS2$[0 0 0]$CS1$CS1$m$[0 0 0]$Euler X-Y-Z$deg$WORLD$true$none  CGPos=[0 0 0]  CGRot=[0 0 0]  CS0Pos=[]  CS0Rot=[]  CS1Pos=[0 0 0]  CS1Rot=[0 0 0]  CS2Pos=[0 0 0]  CS2Rot=[0 0 0]  CS3Pos=[]  CS3Rot=[]  CS4Pos=[]  CS4Rot=[]  CS5Pos=[]  CS5Rot=[]  CS6Pos=[]  CS6Rot=[]  CS7Pos=[]  CS7Rot=[]  CS8Pos=[]  CS8Rot=[]  CS9Pos=[]  CS9Rot=[]  CS10Pos=[]  CS10Rot=[]  CS11Pos=[]  CS11Rot=[]  CS12Pos=[]  CS12Rot=[]  CS13Pos=[]  CS13Rot=[]  CS14Pos=[]  CS14Rot=[]  CS15Pos=[]  CS15Rot=[]  CS16Pos=[]  CS16Rot=[]  CS17Pos=[]  CS17Rot=[]  CS18Pos=[]  CS18Rot=[]  CS19Pos=[]  CS19Rot=[]  CS20Pos=[]  CS20Rot=[]
  Weld1 : mblibv1/Joints/Weld  LConnTagsString=__newl0  RConnTagsString=__newr0  UpdateFromCAD=off  NumSAPorts=0  CutJoint=off  MarkAsCut=off  Primitives=weld  PrimitiveProps=W$World$[0 0 0]$weld  DialogClass=JointBlock  WAxis=[0 0 0]
  to_rev : PMIOPort  Port=1  Side=Right
  to_frame : PMIOPort  Port=2  Side=Left
  connections:
  Body1/LConn1 -- Weld1/RConn1
  to_rev/RConn1 -- Body1/RConn1
  to_frame/RConn1 -- Weld1/LConn1

== system WaterRunner_lib/motor1/motor_body ==
  Body1 : mblibv1/Bodies/Body  LConnTagsString=CS1  RConnTagsString=CS2  UpdateFromCAD=off  DialogClass=MechanicalBodyBlock  Mass=motor_mass  MassUnits=kg  InertiaUnits=kg*m^2  Inertia=motor_inertia  Shape=Cylinder  ShapeDims=[1 1]  ShapeUnits=m  ShapeUse=false  Density=1  DensityUnits=kg/m^3  DensityUse=false  GraphicsMode=CONVHULL  BodyColorSelMode=COLORPALETTE  BodyColor=[0.87059 0.4902 0]  AttachedToCS=CG  CG=Left$CG$[0 0 0]$CS1$CS1$m$[0 0 0]$Euler X-Y-Z$deg$WORLD$false$none  WorkingFrames=Left$CS1$[0 0 0]$Adjoining$Adjoining$m$[0 0 0]$Euler X-Y-Z$deg$WORLD$true$none#Right$CS2$[0 0 0]$CS1$CS1$m$[0 0 0]$Euler X-Y-Z$deg$WORLD$true$none  CGPos=[0 0 0]  CGRot=[0 0 0]  CS0Pos=[]  CS0Rot=[]  CS1Pos=[0 0 0]  CS1Rot=[0 0 0]  CS2Pos=[0 0 0]  CS2Rot=[0 0 0]  CS3Pos=[]  CS3Rot=[]  CS4Pos=[]  CS4Rot=[]  CS5Pos=[]  CS5Rot=[]  CS6Pos=[]  CS6Rot=[]  CS7Pos=[]  CS7Rot=[]  CS8Pos=[]  CS8Rot=[]  CS9Pos=[]  CS9Rot=[]  CS10Pos=[]  CS10Rot=[]  CS11Pos=[]  CS11Rot=[]  CS12Pos=[]  CS12Rot=[]  CS13Pos=[]  CS13Rot=[]  CS14Pos=[]  CS14Rot=[]  CS15Pos=[]  CS15Rot=[]  CS16Pos=[]  CS16Rot=[]  CS17Pos=[]  CS17Rot=[]  CS18Pos=[]  CS18Rot=[]  CS19Pos=[]  CS19Rot=[]  CS20Pos=[]  CS20Rot=[]
  Weld1 : mblibv1/Joints/Weld  LConnTagsString=__newl0  RConnTagsString=__newr0  UpdateFromCAD=off  NumSAPorts=0  CutJoint=off  MarkAsCut=off  Primitives=weld  PrimitiveProps=W$World$[0 0 0]$weld  DialogClass=JointBlock  WAxis=[0 0 0]
  to_rev : PMIOPort  Port=1  Side=Right
  to_frame : PMIOPort  Port=2  Side=Left
  connections:
  to_frame/RConn1 -- Weld1/LConn1
  to_rev/RConn1 -- Body1/RConn1
  Body1/LConn1 -- Weld1/RConn1

== system WaterRunner_lib/servo/motor_body ==
  Body1 : mblibv1/Bodies/Body  LConnTagsString=CS1  RConnTagsString=CS2  UpdateFromCAD=off  DialogClass=MechanicalBodyBlock  Mass=motor_mass  MassUnits=kg  InertiaUnits=kg*m^2  Inertia=motor_inertia  Shape=Cylinder  ShapeDims=[1 1]  ShapeUnits=m  ShapeUse=false  Density=1  DensityUnits=kg/m^3  DensityUse=false  GraphicsMode=CONVHULL  BodyColorSelMode=COLORPALETTE  BodyColor=[0.87059 0.4902 0]  AttachedToCS=CG  CG=Left$CG$[0 0 0]$CS1$CS1$m$[0 0 0]$Euler X-Y-Z$deg$WORLD$false$none  WorkingFrames=Left$CS1$[0 0 0]$Adjoining$Adjoining$m$[0 0 0]$Euler X-Y-Z$deg$WORLD$true$none#Right$CS2$[0 0 0]$CS1$CS1$m$[0 0 0]$Euler X-Y-Z$deg$WORLD$true$none  CGPos=[0 0 0]  CGRot=[0 0 0]  CS0Pos=[]  CS0Rot=[]  CS1Pos=[0 0 0]  CS1Rot=[0 0 0]  CS2Pos=[0 0 0]  CS2Rot=[0 0 0]  CS3Pos=[]  CS3Rot=[]  CS4Pos=[]  CS4Rot=[]  CS5Pos=[]  CS5Rot=[]  CS6Pos=[]  CS6Rot=[]  CS7Pos=[]  CS7Rot=[]  CS8Pos=[]  CS8Rot=[]  CS9Pos=[]  CS9Rot=[]  CS10Pos=[]  CS10Rot=[]  CS11Pos=[]  CS11Rot=[]  CS12Pos=[]  CS12Rot=[]  CS13Pos=[]  CS13Rot=[]  CS14Pos=[]  CS14Rot=[]  CS15Pos=[]  CS15Rot=[]  CS16Pos=[]  CS16Rot=[]  CS17Pos=[]  CS17Rot=[]  CS18Pos=[]  CS18Rot=[]  CS19Pos=[]  CS19Rot=[]  CS20Pos=[]  CS20Rot=[]
  Weld1 : mblibv1/Joints/Weld  LConnTagsString=__newl0  RConnTagsString=__newr0  UpdateFromCAD=off  NumSAPorts=0  CutJoint=off  MarkAsCut=off  Primitives=weld  PrimitiveProps=W$World$[0 0 0]$weld  DialogClass=JointBlock  WAxis=[0 0 0]
  to_rev : PMIOPort  Port=1  Side=Right
  to_frame : PMIOPort  Port=2  Side=Left
  connections:
  to_frame/RConn1 -- Weld1/LConn1
  to_rev/RConn1 -- Body1/RConn1
  Body1/LConn1 -- Weld1/RConn1

== matlab function Tail Pad/MATLAB Function ==
  data: u input double; y output double
function y = fcn(u)
%#codegen
    theta = atan2(u(11),u(10));
    
y = theta;

== matlab function Water Foot/MATLAB Function ==
  data: u input double; y output double
function y = fcn(u)
%#codegen
    theta = -1*atan2(u(11),u(10));
    
y = theta;
